simulink model "segwaycontroller"  (R2016b)
settings: Solver=VariableStepAuto  StartTime=0.0  StopTime=10.0  RelTol=1e-3
libraries: fuzblock x1
settings Model: Creator=nila  LastModifiedBy=nila

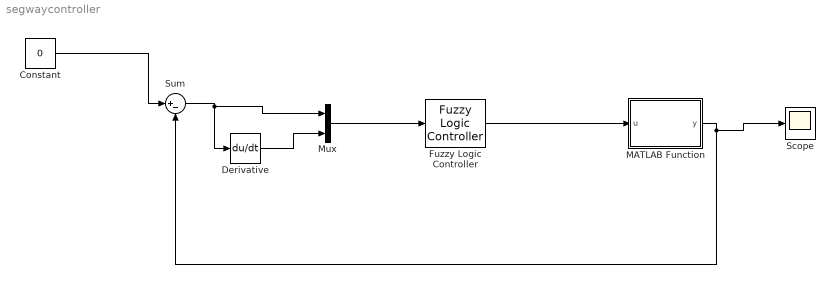
== system segwaycontroller ==
  Constant : Constant  Value=0
  Derivative : Derivative
  Fuzzy Logic Controller : fuzblock/Fuzzy Logic  Controller  fis=segwaycontroler.fis
  MATLAB Function : MATLAB Function  TreatAsAtomicUnit=on
  Mux : Mux  Inputs=2
  Scope : Scope
  Sum : Sum  Inputs=|+-
  wires:
  Constant/1 -> Sum/1
  Mux/1 -> Fuzzy Logic Controller/1
  Sum/1 -> Mux/1, Derivative/1
  Derivative/1 -> Mux/2
  Fuzzy Logic Controller/1 -> MATLAB Function/1(u)
  MATLAB Function/1(y) -> Scope/1, Sum/2

== matlab function segwaycontroller/MATLAB Function ==
  data: u input; y output
function y = fcn(u)

y = u;
